simulink model "nonlinear"  (Simulink 8.1)
settings: Solver=ode45  StartTime=0.0  StopTime=50  RelTol=1e-3
settings Model: Creator=dejanira  LastModifiedBy=dejanira
settings DataIOCC: SignalLoggingSaveFormat=Dataset
settings OptimizationCC: ExpressionDepthLimit=128
settings DebuggingCC: FcnCallInpInsideContextMsg=EnableAllAsError
settings GRTTargetCC: CombineOutputUpdateFcns=on  GRTInterface=off

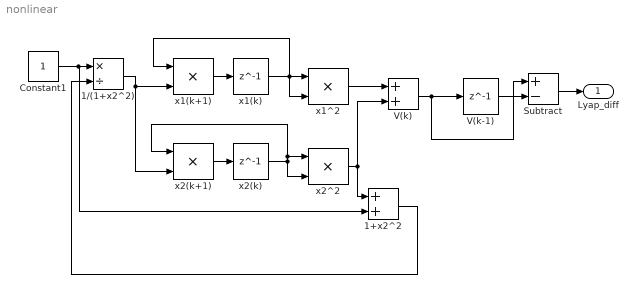
== system nonlinear ==
  1+x2^2 : Sum
  1/(1+x2^2) : Product  Inputs=*/
  Constant1 : Constant
  Subtract : Sum  Inputs=+-
  V(k) : Sum
  V(k-1) : Delay  DelayLength=1  InitialCondition=1000  SampleTime=0.01
  x1(k) : Delay  DelayLength=1
  x1(k+1) : Product  SampleTime=0.1
  x1^2 : Product  SampleTime=0.1
  x2(k) : Delay  DelayLength=1
  x2(k+1) : Product  SampleTime=0.1
  x2^2 : Product  SampleTime=0.1
  Lyap_diff : Outport
  wires:
  x2(k)/1 -> x2(k+1)/1, x2^2/1, x2^2/2
  Constant1/1 -> 1+x2^2/2, 1/(1+x2^2)/1
  x2^2/1 -> 1+x2^2/1, V(k)/2
  1+x2^2/1 -> 1/(1+x2^2)/2
  1/(1+x2^2)/1 -> x1(k+1)/2, x2(k+1)/2
  x1(k)/1 -> x1(k+1)/1, x1^2/1, x1^2/2
  x1^2/1 -> V(k)/1
  V(k-1)/1 -> Subtract/2
  Subtract/1 -> Lyap_diff/1
  V(k)/1 -> V(k-1)/1, Subtract/1
  x1(k+1)/1 -> x1(k)/1
  x2(k+1)/1 -> x2(k)/1
